simulink model "FourCh_TDPA_TD"  (R2021b)
settings: Solver=FixedStepAuto  StartTime=0.0  StopTime=50  FixedStep=0.001  RelTol=1e-3
settings Model: Creator=lucao  LastModifiedBy=lucao

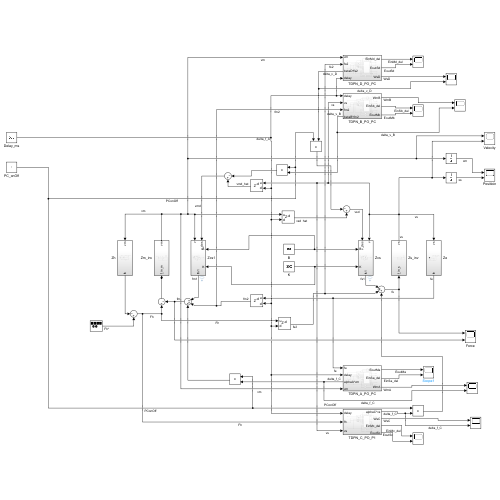
[thumbnail: Simulink's stored preview of the top-level diagram]
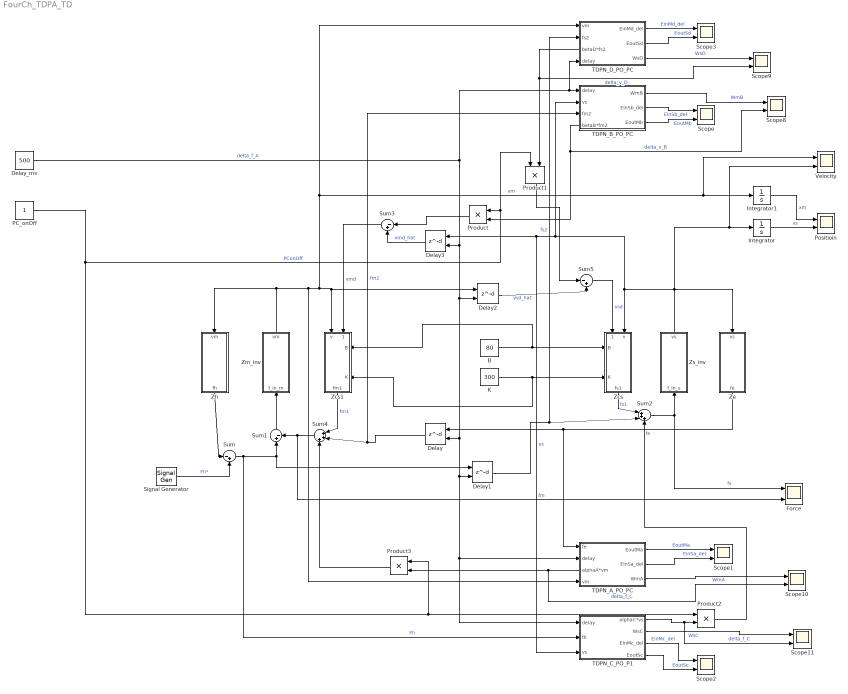
== system FourCh_TDPA_TD ==
  B : Constant  Value=80
  Delay{,1..3} (4 alike) : Delay  DelayLengthSource=Input port  DelayLengthUpperLimit=10000
      settings: InputPortMap=u0,p1
  Delay_ms : Constant  Value=500
  Force : Scope  NumInputPorts=2
  Integrator : Integrator
  Integrator1 : Integrator
  K : Constant  Value=300
  PC_onOff : Constant
  Positioin : Scope  NumInputPorts=2
  Product{,1..3} (4 alike) : Product
  Scope{,1..3,8..11} (8 alike) : Scope  NumInputPorts=2
  Signal Generator : SignalGenerator  Amplitude=10  Frequency=0.25
  Sum : Sum  Inputs=|-+
  Sum1 : Sum  Inputs=|+-
  Sum2 : Sum  Inputs=|+++
  Sum3 : Sum  Inputs=|-+
  Sum4 : Sum  Inputs=|+++
  Sum5 : Sum  Inputs=|-+
  TDPN_A_PO_PC : Subsystem
      settings: PortSchema="{\"entries\":[{\"content\":{\"sides\":[{\"content\":{\"connectorIds\":[\"In1\",\"In2\",\"Out4\",\"In3\"]},\"type\":\"ConnectorPlacement.EquallySpacedRectSide\",\"uuid\":\"a886a96f-0c36-41e2-9566-9e512c297510\"},{\"content\":{\"connectorIds\":[\"Out1\",\"Out2\",\"Out3\"],\"side\":\"RIGHT\"},\"type\":\"ConnectorPlacement.EquallySpacedRectSide\",\"uuid\":\"ded73008-176a-40b3-991c-7df602be33ae\"},{\"content\":{\"connectorIds\":[],\"side\":\"TOP\"},\"type\":\"ConnectorPlacement.EquallySpacedRectSide\",\"uuid\":\"df3bf8a9-b958-40b3-ae2e-9520b93dbcdb\"}]},\"type\":\"ConnectorPlacement.EquallySpacedConnector\",\"uuid\":\"1b05d7b7-d9bf-444b-93d4-0d97d5e5cfa2\"}],\"packageUris\":[\"http://schema.mathworks.com/mf0/Connector/R2020b\"],\"version\":\"1.0\"}"
  TDPN_B_PO_PC : Subsystem
      settings: PortSchema="{\"entries\":[{\"content\":{\"sides\":[{\"content\":{\"connectorIds\":[\"In1\",\"In2\",\"In3\",\"Out4\"]},\"type\":\"ConnectorPlacement.EquallySpacedRectSide\",\"uuid\":\"a886a96f-0c36-41e2-9566-9e512c297510\"},{\"content\":{\"connectorIds\":[\"Out1\",\"Out2\",\"Out3\"],\"side\":\"RIGHT\"},\"type\":\"ConnectorPlacement.EquallySpacedRectSide\",\"uuid\":\"ded73008-176a-40b3-991c-7df602be33ae\"},{\"content\":{\"connectorIds\":[],\"side\":\"TOP\"},\"type\":\"ConnectorPlacement.EquallySpacedRectSide\",\"uuid\":\"df3bf8a9-b958-40b3-ae2e-9520b93dbcdb\"}]},\"type\":\"ConnectorPlacement.EquallySpacedConnector\",\"uuid\":\"1b05d7b7-d9bf-444b-93d4-0d97d5e5cfa2\"}],\"packageUris\":[\"http://schema.mathworks.com/mf0/Connector/R2020b\"],\"version\":\"1.0\"}"
  TDPN_C_PO_P1 : Subsystem
  TDPN_D_PO_PC : Subsystem
      settings: PortSchema="{\"entries\":[{\"content\":{\"sides\":[{\"content\":{\"connectorIds\":[\"In1\",\"In2\",\"Out4\",\"In3\"]},\"type\":\"ConnectorPlacement.EquallySpacedRectSide\",\"uuid\":\"a886a96f-0c36-41e2-9566-9e512c297510\"},{\"content\":{\"connectorIds\":[\"Out1\",\"Out2\",\"Out3\"],\"side\":\"RIGHT\"},\"type\":\"ConnectorPlacement.EquallySpacedRectSide\",\"uuid\":\"ded73008-176a-40b3-991c-7df602be33ae\"},{\"content\":{\"connectorIds\":[],\"side\":\"TOP\"},\"type\":\"ConnectorPlacement.EquallySpacedRectSide\",\"uuid\":\"df3bf8a9-b958-40b3-ae2e-9520b93dbcdb\"}]},\"type\":\"ConnectorPlacement.EquallySpacedConnector\",\"uuid\":\"1b05d7b7-d9bf-444b-93d4-0d97d5e5cfa2\"}],\"packageUris\":[\"http://schema.mathworks.com/mf0/Connector/R2020b\"],\"version\":\"1.0\"}"
  Velocity : Scope  NumInputPorts=2
  Zcs : Subsystem
      settings: PortSchema="{\"entries\":[{\"content\":{\"sides\":[{\"content\":{\"connectorIds\":[\"In1\",\"In2\"]},\"type\":\"ConnectorPlacement.EquallySpacedRectSide\",\"uuid\":\"c32e4091-a441-4f3b-b0b8-cebe01d42adf\"},{\"content\":{\"connectorIds\":[\"Out1\"],\"side\":\"RIGHT\"},\"type\":\"ConnectorPlacement.EquallySpacedRectSide\",\"uuid\":\"ccadc46e-4cdd-4994-a822-3ba84443801c\"},{\"content\":{\"connectorIds\":[\"In3\",\"In4\"],\"side\":\"TOP\"},\"type\":\"ConnectorPlacement.EquallySpacedRectSide\",\"uuid\":\"020656f3-557f-4da7-a585-94cb368715db\"}]},\"type\":\"ConnectorPlacement.EquallySpacedConnector\",\"uuid\":\"4a9455fd-3018-4498-b276-9155c948801a\"}],\"packageUris\":[\"http://schema.mathworks.com/mf0/Connector/R2020b\"],\"version\":\"1.0\"}"
  Zcs1 : Subsystem
      settings: PortSchema="{\"entries\":[{\"content\":{\"sides\":[{\"content\":{\"connectorIds\":[\"In1\",\"In2\"]},\"type\":\"ConnectorPlacement.EquallySpacedRectSide\",\"uuid\":\"c32e4091-a441-4f3b-b0b8-cebe01d42adf\"},{\"content\":{\"connectorIds\":[\"Out1\"],\"side\":\"RIGHT\"},\"type\":\"ConnectorPlacement.EquallySpacedRectSide\",\"uuid\":\"ccadc46e-4cdd-4994-a822-3ba84443801c\"},{\"content\":{\"connectorIds\":[\"In3\",\"In4\"],\"side\":\"TOP\"},\"type\":\"ConnectorPlacement.EquallySpacedRectSide\",\"uuid\":\"020656f3-557f-4da7-a585-94cb368715db\"}]},\"type\":\"ConnectorPlacement.EquallySpacedConnector\",\"uuid\":\"4a9455fd-3018-4498-b276-9155c948801a\"}],\"packageUris\":[\"http://schema.mathworks.com/mf0/Connector/R2020b\"],\"version\":\"1.0\"}"
  Ze : Subsystem
  Zh : Subsystem
  Zm_inv : Subsystem
  Zs_inv : Subsystem
  wires:
  Zm_inv/1(vm) -> Zh/1(vm), TDPN_A_PO_PC/3(vm), TDPN_D_PO_PC/1(vm), Velocity/1, Integrator1/1, Delay2/1, Zcs1/2(v)  "vm"
  Zh/1(fh) -> Sum/1
  Ze/1(fe) -> TDPN_A_PO_PC/1(fe), Delay/1  "fe"
  Sum1/1 -> Zm_inv/1(f_in_m)
  Zcs/1(fs1) -> Sum2/1  "fs1"
  Zs_inv/1(vs) -> Velocity/2, Integrator/1, Delay3/1, TDPN_C_PO_P1/3(vs), TDPN_B_PO_PC/2(vs), Zcs/2(v), Ze/1(vs)  "vs"
  Integrator/1 -> Positioin/2  "xs"
  Signal Generator/1 -> Sum/2  "Fh*"
  Sum2/1 -> Force/1, Zs_inv/1(f_in_s)  "fs"
  Sum/1 -> TDPN_C_PO_P1/2(fh), Sum1/1, Delay1/1  "Fh"
  K/1 -> Zcs1/4(K), Zcs/4(K)
  B/1 -> Zcs1/3(B), Zcs/3(B)
  Integrator1/1 -> Positioin/1  "xm"
  Zcs1/1(fm1) -> Sum4/1  "fm1"
  Delay/1 -> TDPN_B_PO_PC/3(fm2), Sum4/2  "fm2"
  Sum4/1 -> Force/2, Sum1/2  "fm"
  Delay1/1 -> TDPN_D_PO_PC/2(fs2), Sum2/2  "fs2"
  Delay3/1 -> Sum3/2  "vmd_hat"
  Sum3/1 -> Zcs1/1(v_des)  "vmd"
  Delay_ms/1 -> Delay3/2, Delay2/2, Delay1/2, TDPN_C_PO_P1/1(delay), TDPN_A_PO_PC/2(delay), Delay/2, TDPN_D_PO_PC/3(delay), TDPN_B_PO_PC/1(delay)  "delta_f_A"
  Sum5/1 -> Zcs/1(v_des)  "vsd"
  Delay2/1 -> Sum5/2  "vsd_hat"
  TDPN_B_PO_PC/4(betaB*fm2) -> Scope8/2, Product/2  "delta_v_B"
  Product/1 -> Sum3/1
  PC_onOff/1 -> Product3/1, Product2/1, Product1/1, Product/1  "PConOff"
  TDPN_D_PO_PC/4(betaD*fs2) -> Scope9/2, Product1/2  "delta_v_D"
  Product1/1 -> Sum5/1
  TDPN_C_PO_P1/1(alphaC*vs) -> Scope11/2, Product2/2  "delta_f_C"
  Product2/1 -> Sum2/3
  TDPN_A_PO_PC/4(alphaA*vm) -> Scope10/2, Product3/2  "delta_f_C"
  Product3/1 -> Sum4/3
  TDPN_A_PO_PC/1(EoutMa) -> Scope1/1  "EoutMa"
  TDPN_A_PO_PC/2(EinSa_del) -> Scope1/2  "EinSa_del"
  TDPN_C_PO_P1/3(EinMc_del) -> Scope2/1  "EinMc_del"
  TDPN_C_PO_P1/4(EoutSc) -> Scope2/2  "EoutSc"
  TDPN_B_PO_PC/2(EinSb_del) -> Scope/1  "EinSb_del"
  TDPN_B_PO_PC/3(EoutMb) -> Scope/2  "EoutMb"
  TDPN_D_PO_PC/2(EoutSd) -> Scope3/2  "EoutSd"
  TDPN_D_PO_PC/1(EinMd_del) -> Scope3/1  "EinMd_del"
  TDPN_B_PO_PC/1(WmB) -> Scope8/1  "WmB"
  TDPN_D_PO_PC/3(WsD) -> Scope9/1  "WsD"
  TDPN_A_PO_PC/3(WmA) -> Scope10/1  "WmA"
  TDPN_C_PO_P1/2(WsC) -> Scope11/1  "WsC"

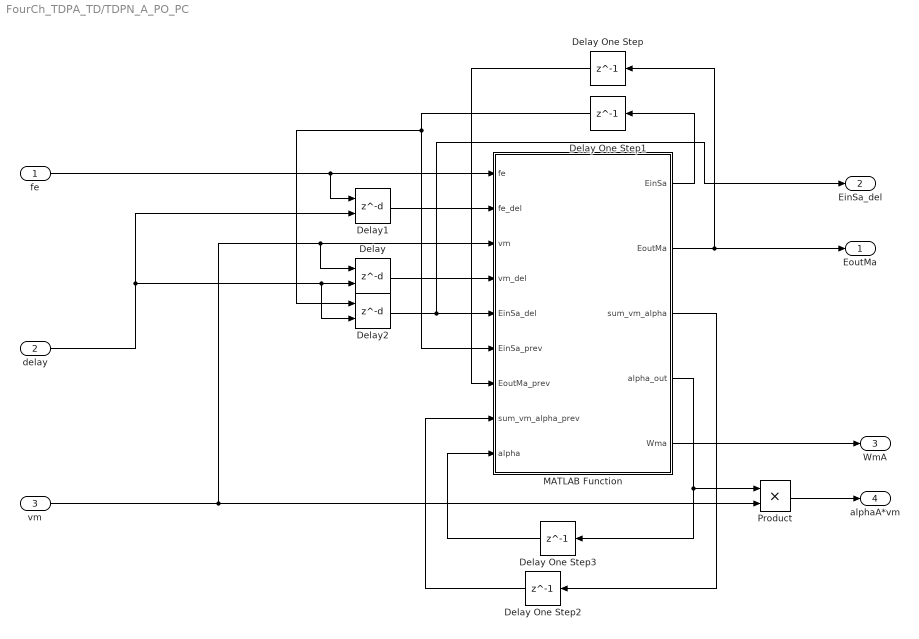
== system FourCh_TDPA_TD/TDPN_A_PO_PC ==
  fe : Inport
  delay : Inport  Port=2
  vm : Inport  Port=3
  Delay : Delay  DelayLengthSource=Input port  DelayLengthUpperLimit=10000
      settings: InputPortMap=u0,p1
  Delay One Step{,1..3} (4 alike) : Delay  DelayLength=1
  Delay1 : Delay  DelayLengthSource=Input port  DelayLengthUpperLimit=10000
      settings: InputPortMap=u0,p1
  Delay2 : Delay  DelayLengthSource=Input port  DelayLengthUpperLimit=10000
      settings: InputPortMap=u0,p1
  MATLAB Function : MATLAB Function  TreatAsAtomicUnit=on
  Product : Product
  EoutMa : Outport
  EinSa_del : Outport  Port=2
  WmA : Outport  Port=3
  alphaA*vm : Outport  Port=4
  wires:
  Product/1 -> alphaA*vm/1
  MATLAB Function/4(alpha_out) -> Product/1, Delay One Step3/1
  vm/1 -> Product/2, Delay/1, MATLAB Function/3(vm)
  delay/1 -> Delay1/2, Delay2/2, Delay/2
  Delay/1 -> MATLAB Function/4(vm_del)
  fe/1 -> Delay1/1, MATLAB Function/1(fe)
  Delay1/1 -> MATLAB Function/2(fe_del)
  MATLAB Function/1(EinSa) -> Delay One Step1/1
  Delay2/1 -> EinSa_del/1, MATLAB Function/5(EinSa_del)
  MATLAB Function/2(EoutMa) -> Delay One Step/1, EoutMa/1
  MATLAB Function/3(sum_vm_alpha) -> Delay One Step2/1
  Delay One Step/1 -> MATLAB Function/7(EoutMa_prev)
  Delay One Step1/1 -> MATLAB Function/6(EinSa_prev), Delay2/1
  Delay One Step2/1 -> MATLAB Function/8(sum_vm_alpha_prev)
  Delay One Step3/1 -> MATLAB Function/9(alpha)
  MATLAB Function/5(Wma) -> WmA/1

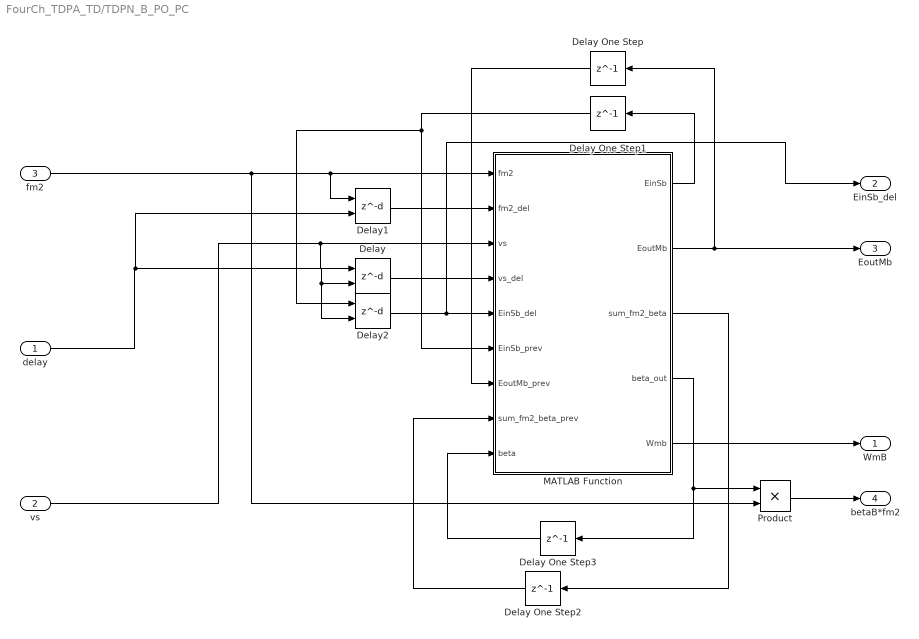
== system FourCh_TDPA_TD/TDPN_B_PO_PC ==
  delay : Inport
  vs : Inport  Port=2
  fm2 : Inport  Port=3
  Delay : Delay  DelayLengthSource=Input port  DelayLengthUpperLimit=10000
      settings: InputPortMap=u0,p1
  Delay One Step{,1..3} (4 alike) : Delay  DelayLength=1
  Delay1 : Delay  DelayLengthSource=Input port  DelayLengthUpperLimit=10000
      settings: InputPortMap=u0,p1
  Delay2 : Delay  DelayLengthSource=Input port  DelayLengthUpperLimit=10000
      settings: InputPortMap=u0,p1
  MATLAB Function : MATLAB Function  TreatAsAtomicUnit=on
  Product : Product
  WmB : Outport
  EinSb_del : Outport  Port=2
  EoutMb : Outport  Port=3
  betaB*fm2 : Outport  Port=4
  wires:
  Product/1 -> betaB*fm2/1
  MATLAB Function/4(beta_out) -> Product/1, Delay One Step3/1
  vs/1 -> Delay/1, MATLAB Function/3(vs)
  delay/1 -> Delay1/2, Delay2/2, Delay/2
  Delay/1 -> MATLAB Function/4(vs_del)
  fm2/1 -> Product/2, Delay1/1, MATLAB Function/1(fm2)
  Delay1/1 -> MATLAB Function/2(fm2_del)
  MATLAB Function/1(EinSb) -> Delay One Step1/1
  Delay2/1 -> EinSb_del/1, MATLAB Function/5(EinSb_del)
  MATLAB Function/2(EoutMb) -> EoutMb/1, Delay One Step/1
  MATLAB Function/3(sum_fm2_beta) -> Delay One Step2/1
  Delay One Step/1 -> MATLAB Function/7(EoutMb_prev)
  Delay One Step1/1 -> MATLAB Function/6(EinSb_prev), Delay2/1
  Delay One Step2/1 -> MATLAB Function/8(sum_fm2_beta_prev)
  Delay One Step3/1 -> MATLAB Function/9(beta)
  MATLAB Function/5(Wmb) -> WmB/1

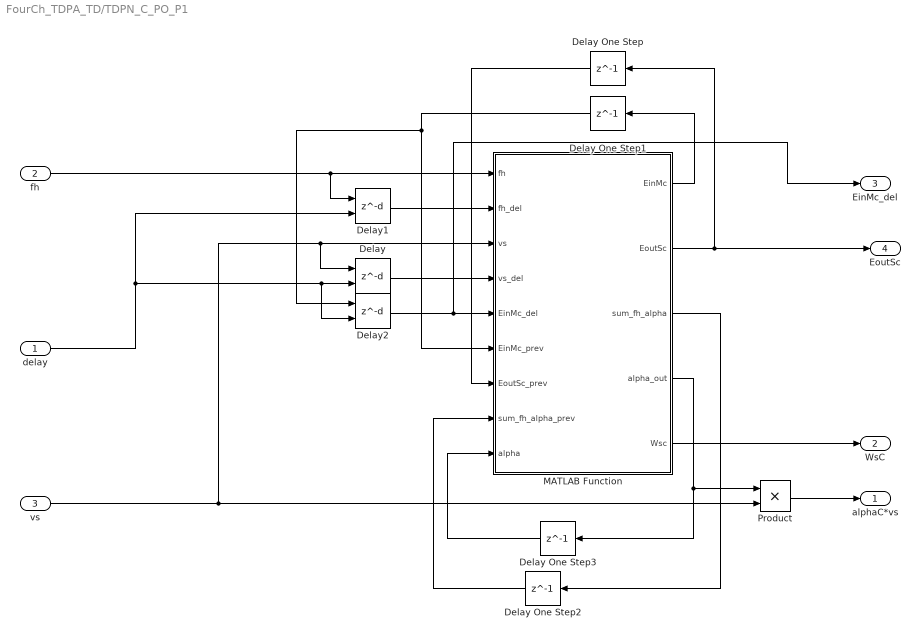
== system FourCh_TDPA_TD/TDPN_C_PO_P1 ==
  delay : Inport
  fh : Inport  Port=2
  vs : Inport  Port=3
  Delay : Delay  DelayLengthSource=Input port  DelayLengthUpperLimit=10000
      settings: InputPortMap=u0,p1
  Delay One Step{,1..3} (4 alike) : Delay  DelayLength=1
  Delay1 : Delay  DelayLengthSource=Input port  DelayLengthUpperLimit=10000
      settings: InputPortMap=u0,p1
  Delay2 : Delay  DelayLengthSource=Input port  DelayLengthUpperLimit=10000
      settings: InputPortMap=u0,p1
  MATLAB Function : MATLAB Function  TreatAsAtomicUnit=on
  Product : Product
  alphaC*vs : Outport
  WsC : Outport  Port=2
  EinMc_del : Outport  Port=3
  EoutSc : Outport  Port=4
  wires:
  Product/1 -> alphaC*vs/1
  MATLAB Function/4(alpha_out) -> Product/1, Delay One Step3/1
  vs/1 -> Product/2, Delay/1, MATLAB Function/3(vs)
  delay/1 -> Delay1/2, Delay2/2, Delay/2
  Delay/1 -> MATLAB Function/4(vs_del)
  fh/1 -> Delay1/1, MATLAB Function/1(fh)
  Delay1/1 -> MATLAB Function/2(fh_del)
  MATLAB Function/1(EinMc) -> Delay One Step1/1
  Delay2/1 -> EinMc_del/1, MATLAB Function/5(EinMc_del)
  MATLAB Function/2(EoutSc) -> EoutSc/1, Delay One Step/1
  MATLAB Function/3(sum_fh_alpha) -> Delay One Step2/1
  Delay One Step/1 -> MATLAB Function/7(EoutSc_prev)
  Delay One Step1/1 -> MATLAB Function/6(EinMc_prev), Delay2/1
  Delay One Step2/1 -> MATLAB Function/8(sum_fh_alpha_prev)
  Delay One Step3/1 -> MATLAB Function/9(alpha)
  MATLAB Function/5(Wsc) -> WsC/1

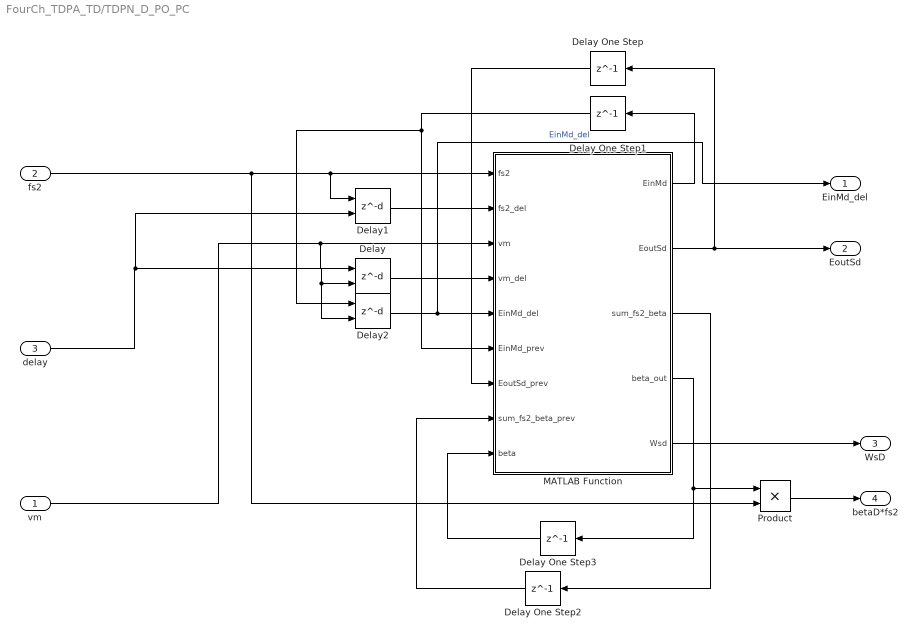
== system FourCh_TDPA_TD/TDPN_D_PO_PC ==
  vm : Inport
  fs2 : Inport  Port=2
  delay : Inport  Port=3
  Delay : Delay  DelayLengthSource=Input port  DelayLengthUpperLimit=10000
      settings: InputPortMap=u0,p1
  Delay One Step{,1..3} (4 alike) : Delay  DelayLength=1
  Delay1 : Delay  DelayLengthSource=Input port  DelayLengthUpperLimit=10000
      settings: InputPortMap=u0,p1
  Delay2 : Delay  DelayLengthSource=Input port  DelayLengthUpperLimit=10000
      settings: InputPortMap=u0,p1
  MATLAB Function : MATLAB Function  TreatAsAtomicUnit=on
  Product : Product
  EinMd_del : Outport
  EoutSd : Outport  Port=2
  WsD : Outport  Port=3
  betaD*fs2 : Outport  Port=4
  wires:
  Product/1 -> betaD*fs2/1
  MATLAB Function/4(beta_out) -> Product/1, Delay One Step3/1
  vm/1 -> Delay/1, MATLAB Function/3(vm)
  delay/1 -> Delay1/2, Delay2/2, Delay/2
  Delay/1 -> MATLAB Function/4(vm_del)
  fs2/1 -> Product/2, Delay1/1, MATLAB Function/1(fs2)
  Delay1/1 -> MATLAB Function/2(fs2_del)
  MATLAB Function/1(EinMd) -> Delay One Step1/1
  MATLAB Function/2(EoutSd) -> EoutSd/1, Delay One Step/1
  MATLAB Function/3(sum_fs2_beta) -> Delay One Step2/1
  Delay One Step/1 -> MATLAB Function/7(EoutSd_prev)
  Delay One Step1/1 -> MATLAB Function/6(EinMd_prev), Delay2/1
  Delay One Step2/1 -> MATLAB Function/8(sum_fs2_beta_prev)
  Delay One Step3/1 -> MATLAB Function/9(beta)
  MATLAB Function/5(Wsd) -> WsD/1
  Delay2/1 -> EinMd_del/1, MATLAB Function/5(EinMd_del)  "EinMd_del"

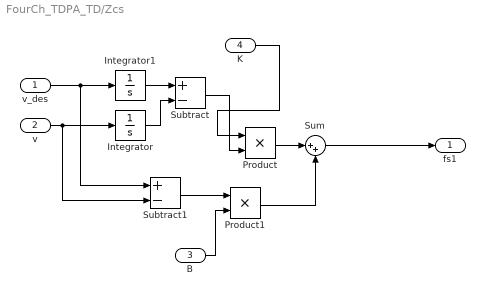
== system FourCh_TDPA_TD/Zcs ==
  v_des : Inport
  v : Inport  Port=2
  B : Inport  Port=3
  K : Inport  Port=4
  Integrator : Integrator
  Integrator1 : Integrator
  Product : Product
  Product1 : Product
  Subtract : Sum  Inputs=+-
  Subtract1 : Sum  Inputs=+-
  Sum : Sum  Inputs=|++
  fs1 : Outport
  wires:
  v_des/1 -> Integrator1/1, Subtract1/1
  v/1 -> Subtract1/2, Integrator/1
  Subtract/1 -> Product/2
  Subtract1/1 -> Product1/1
  Product/1 -> Sum/1
  Product1/1 -> Sum/2
  Sum/1 -> fs1/1
  Integrator/1 -> Subtract/2
  Integrator1/1 -> Subtract/1
  K/1 -> Product/1
  B/1 -> Product1/2

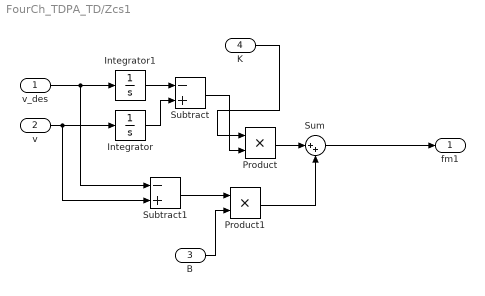
== system FourCh_TDPA_TD/Zcs1 ==
  v_des : Inport
  v : Inport  Port=2
  B : Inport  Port=3
  K : Inport  Port=4
  Integrator : Integrator
  Integrator1 : Integrator
  Product : Product
  Product1 : Product
  Subtract : Sum  Inputs=-+
  Subtract1 : Sum  Inputs=-+
  Sum : Sum  Inputs=|++
  fm1 : Outport
  wires:
  v_des/1 -> Integrator1/1, Subtract1/1
  v/1 -> Subtract1/2, Integrator/1
  Subtract/1 -> Product/2
  Subtract1/1 -> Product1/1
  Product/1 -> Sum/1
  Product1/1 -> Sum/2
  Sum/1 -> fm1/1
  Integrator/1 -> Subtract/2
  Integrator1/1 -> Subtract/1
  K/1 -> Product/1
  B/1 -> Product1/2

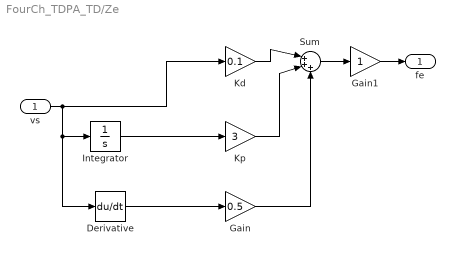
== system FourCh_TDPA_TD/Ze ==
  vs : Inport
  Derivative : Derivative
  Gain : Gain  Gain=0.5
  Gain1 : Gain
  Integrator : Integrator
  Kd : Gain  Gain=0.1
  Kp : Gain  Gain=3
  Sum : Sum  Inputs=|+++
  fe : Outport
  wires:
  vs/1 -> Derivative/1, Integrator/1, Kd/1
  Kp/1 -> Sum/2
  Kd/1 -> Sum/1
  Sum/1 -> Gain1/1
  Gain/1 -> Sum/3
  Gain1/1 -> fe/1
  Integrator/1 -> Kp/1
  Derivative/1 -> Gain/1

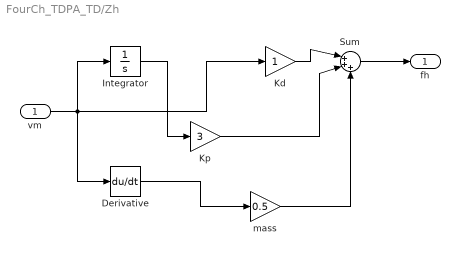
== system FourCh_TDPA_TD/Zh ==
  vm : Inport
  Derivative : Derivative
  Integrator : Integrator
  Kd : Gain
  Kp : Gain  Gain=3
  Sum : Sum  Inputs=|+++
  mass : Gain  Gain=0.5
  fh : Outport
  wires:
  Kp/1 -> Sum/2
  Kd/1 -> Sum/1
  Sum/1 -> fh/1
  Integrator/1 -> Kp/1
  Derivative/1 -> mass/1
  mass/1 -> Sum/3
  vm/1 -> Derivative/1, Integrator/1, Kd/1

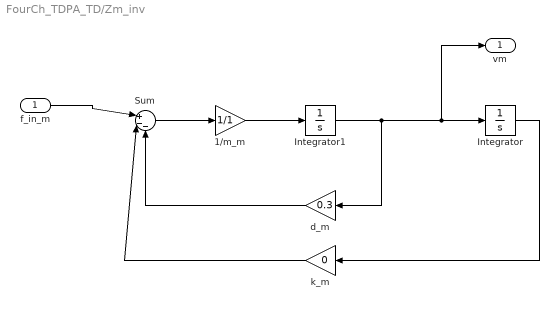
== system FourCh_TDPA_TD/Zm_inv ==
  f_in_m : Inport
  1/m_m : Gain  Gain=1/1
  Integrator : Integrator
  Integrator1 : Integrator
  Sum : Sum  Inputs=|+--
  d_m : Gain  Gain=0.3
  k_m : Gain  Gain=0
  vm : Outport
  wires:
  Integrator/1 -> k_m/1
  Integrator1/1 -> d_m/1, vm/1, Integrator/1
  f_in_m/1 -> Sum/1
  d_m/1 -> Sum/3
  k_m/1 -> Sum/2
  Sum/1 -> 1/m_m/1
  1/m_m/1 -> Integrator1/1

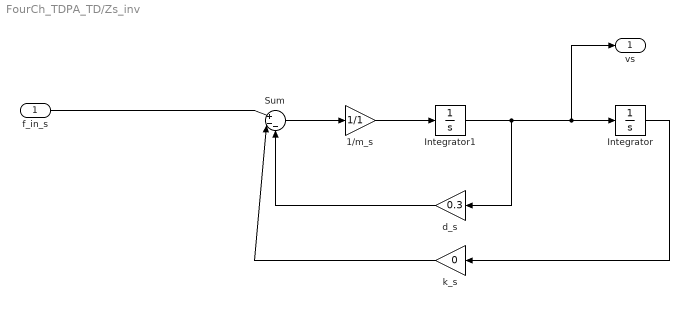
== system FourCh_TDPA_TD/Zs_inv ==
  f_in_s : Inport
  1/m_s : Gain  Gain=1/1
  Integrator : Integrator
  Integrator1 : Integrator
  Sum : Sum  Inputs=|+--
  d_s : Gain  Gain=0.3
  k_s : Gain  Gain=0
  vs : Outport
  wires:
  Integrator/1 -> k_s/1
  Integrator1/1 -> d_s/1, vs/1, Integrator/1
  f_in_s/1 -> Sum/1
  d_s/1 -> Sum/3
  k_s/1 -> Sum/2
  Sum/1 -> 1/m_s/1
  1/m_s/1 -> Integrator1/1

== matlab function FourCh_TDPA_TD/TDPN_B_PO_PC/MATLAB Function ==
  data: fm2 input; EinSb output; fm2_del input; vs input; vs_del input; EinSb_del input; EinSb_prev input; EoutMb_prev input; sum_fm2_beta_prev input; beta input; EoutMb output; sum_fm2_beta output; beta_out output; Wmb output
function [EinSb, EoutMb, sum_fm2_beta, beta_out, Wmb] = fcn(fm2,fm2_del, vs, vs_del, EinSb_del, EinSb_prev, EoutMb_prev,sum_fm2_beta_prev, beta)

    if (-fm2_del*vs>0)
        PinSb = -fm2_del*vs;
    else
        PinSb = 0;
    end
    if (fm2*vs_del<0)
        PoutMb = -fm2*vs_del;
    else
        PoutMb = 0;
    end
    EinSb = EinSb_prev + 0.001*PinSb;
    EoutMb = EoutMb_prev + 0.001*PoutMb;

    EPCMb = 0.001*sum_fm2_beta_prev; 

    Wmb = EinSb_del - EoutMb + EPCMb;

    if (Wmb>0)
        beta_out = 0;
    else
        if (fm2~=0)
            beta_out = -Wmb/(0.001*fm2^2);
        else
            beta_out = 0;
        end
    end

    sum_fm2_beta = sum_fm2_beta_prev + fm2^2*beta;

== matlab function FourCh_TDPA_TD/TDPN_A_PO_PC/MATLAB Function ==
  data: fe input; EinSa output; fe_del input; vm input; vm_del input; EinSa_del input; EinSa_prev input; EoutMa_prev input; sum_vm_alpha_prev input; alpha input; EoutMa output; sum_vm_alpha output; alpha_out output; Wma output
function [EinSa, EoutMa, sum_vm_alpha, alpha_out, Wma] = fcn(fe,fe_del, vm, vm_del, EinSa_del, EinSa_prev, EoutMa_prev, sum_vm_alpha_prev, alpha)

    if (-fe*vm_del>0)
        PinSa = -fe*vm_del;
    else
        PinSa = 0;
    end
    if (fe_del*vm<0)
        PoutMa = -fe_del*vm;
    else
        PoutMa = 0;
    end
    EinSa = EinSa_prev + 0.001*PinSa;
    EoutMa = EoutMa_prev + 0.001*PoutMa;

    EPCMa = 0.001*sum_vm_alpha_prev;

    Wma = EinSa_del - EoutMa + EPCMa;

    if (Wma>0)
        alpha_out = 0;
    else
        if (vm~=0)
            alpha_out = -Wma/(0.001*vm^2);
        else
            alpha_out = 0;
        end
    end
    
    sum_vm_alpha = sum_vm_alpha_prev + vm^2*alpha;

== matlab function FourCh_TDPA_TD/TDPN_C_PO_P1/MATLAB Function ==
  data: fh input; EinMc output; fh_del input; vs input; vs_del input; EinMc_del input; EinMc_prev input; EoutSc_prev input; sum_fh_alpha_prev input; alpha input; EoutSc output; sum_fh_alpha output; alpha_out output; Wsc output
function [EinMc, EoutSc, sum_fh_alpha, alpha_out, Wsc] = fcn(fh,fh_del, vs, vs_del, EinMc_del, EinMc_prev, EoutSc_prev,sum_fh_alpha_prev, alpha)

    if (fh*vs_del>0)
        PinMc = fh*vs_del;
    else
        PinMc = 0;
    end
    if (-fh_del*vs<0)
        PoutSc = fh_del*vs;
    else
        PoutSc = 0;
    end
    EinMc = EinMc_prev + 0.001*PinMc;
    EoutSc = EoutSc_prev + 0.001*PoutSc;

    EPCSc = 0.001*sum_fh_alpha_prev;

    Wsc = EinMc_del - EoutSc + EPCSc;

    if (Wsc>0)
        alpha_out = 0;
    else
        if (vs~=0)
            alpha_out = -Wsc/(0.001*vs^2);
        else
            alpha_out = 0;
        end
    end

    sum_fh_alpha = sum_fh_alpha_prev + vs^2*alpha;

== matlab function FourCh_TDPA_TD/TDPN_D_PO_PC/MATLAB Function ==
  data: fs2 input; EinMd output; fs2_del input; vm input; vm_del input; EinMd_del input; EinMd_prev input; EoutSd_prev input; sum_fs2_beta_prev input; beta input; EoutSd output; sum_fs2_beta output; beta_out output; Wsd output
function [EinMd, EoutSd, sum_fs2_beta, beta_out, Wsd] = fcn(fs2,fs2_del, vm, vm_del, EinMd_del, EinMd_prev, EoutSd_prev,sum_fs2_beta_prev, beta)

    if (fs2_del*vm>0)
        PinMd = fs2_del*vm;
    else
        PinMd = 0;
    end
    if (-fs2*vm_del<0)
        PoutSd = fs2*vm_del;
    else
        PoutSd = 0;
    end
    EinMd = EinMd_prev + 0.001*PinMd;
    EoutSd = EoutSd_prev + 0.001*PoutSd;

    EPCSd = 0.001*sum_fs2_beta_prev;

    Wsd = EinMd_del - EoutSd + EPCSd;

    if (Wsd>0)
        beta_out = 0;
    else
        if (fs2~=0)
            beta_out = -Wsd/(0.001*fs2^2);
        else
            beta_out = 0;
        end
    end

    sum_fs2_beta = sum_fs2_beta_prev+fs2^2*beta;
